simulink model "PE_test"  (R2022b)
settings: Solver=FixedStepAuto  StartTime=0.0  StopTime=50000  FixedStep=0.05  RelTol=1e-13
values from neighbouring files (symbols this model uses):
  A0 = angle2dcm(E1-0.5,E2+0.8,E3+0.3,'ZXY')    [Pointing_tuning.m]
  n = sqrt(settings.mu/settings.a^3)    [Pointing_tuning.m]    (also in control_tuning.m)
undefined symbols (not defined in the file or in its folder): DiscIntNeverNeededParam, environment, r0, sat, settings, thruster, v0
libraries: matrix_library x4, vrlib x4, cstblocks x2
settings Model: SimulationMode=accelerator  Creator=robertopistonenascone  LastModifiedBy=brent

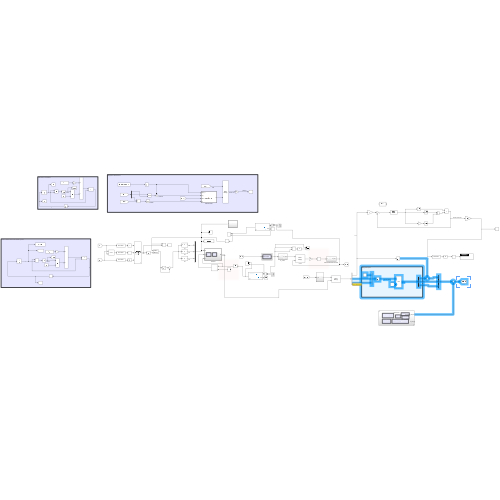
[thumbnail: Simulink's stored preview of the top-level diagram]
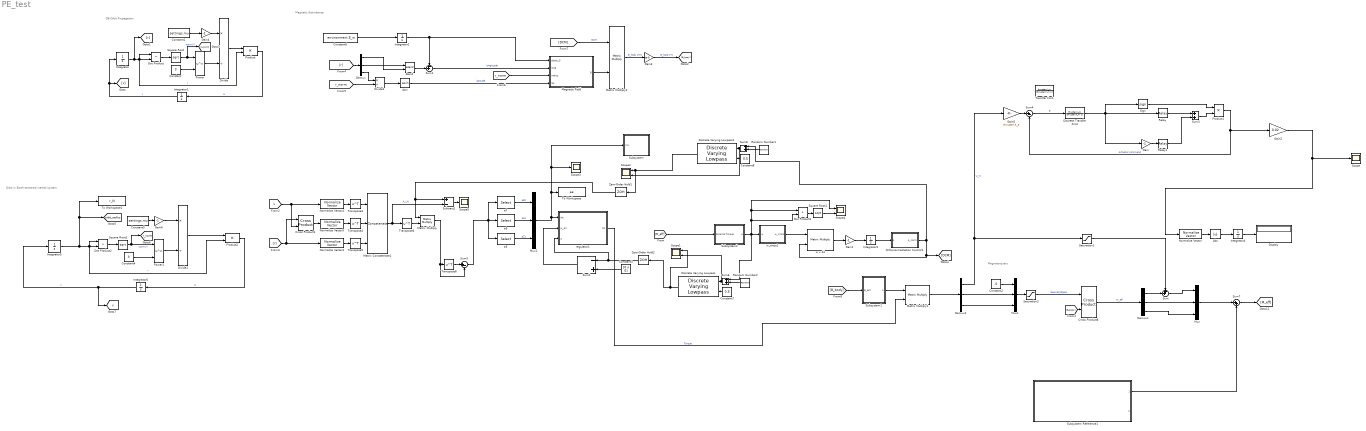
== system PE_test ==
  note: OB Orbit Propagation
  note: Magnetorquers
  note: Magnetic disturbance
  note: Orbit in Earth-centered inertial system
  " w x A1" : Product  Multiplication=Matrix(*)
  Abs : Abs  SaturateOnIntegerOverflow=off
  Asin : Trigonometry  Operator=asin
  Atan2 : Trigonometry  Operator=atan2
  Constant : Constant  Value=3
  Constant1 : Constant  Value=settings.mu
  Constant2 : Constant  Value=0
  Constant3 : Constant  Value=[0 n 0]
  Constant4 : Constant  Value=3
  Constant5 : Constant  Value=settings.mu
  Constant6 : Constant  Value=environment.E_w
  Constant7 : Constant  Value=0.5
  Constant8 : Constant  Value=0.5
  Cross Product1 : matrix_library/Cross Product
  Cross Product8 : matrix_library/Cross Product
  Demux : Demux  Outputs=3
  Demux1 : Demux  Outputs=3
  Demux2 : Demux  Outputs=3
  Discrete Transfer Fcn2 : DiscreteTransferFcn  Numerator=thruster.K_m  Denominator=[thruster.T_m 1]  SampleTime=0.05
  Discrete Varying Lowpass : cstblocks/Linear Parameter Varying/Discrete Varying Lowpass  N=1  w0=0  Ts=0.05
  Discrete Varying Lowpass1 : cstblocks/Linear Parameter Varying/Discrete Varying Lowpass  N=1  w0=0  Ts=0.05
  Display : Display
  Divide : Product  Inputs=*/
  Divide1 : Product  Inputs=*/
  Divide2 : Product  Inputs=*/
  Dot Product : DotProduct  OutDataTypeStr=Inherit: Inherit via internal rule
  Dot Product1 : DotProduct  OutDataTypeStr=Inherit: Inherit via internal rule
  Dot Product2 : DotProduct  OutDataTypeStr=Inherit: Inherit via internal rule
  Gain{,1,4,6} (4 alike) : Gain  Gain=-1
  Gain2 : Gain  Gain=0.02
  Gain3 : Gain  Gain=1e-9
  Gain5 : Gain  Gain=thruster.K_e
  Integrator : Integrator  InitialCondition=r0
  Integrator1 : Integrator  InitialCondition=v0
  Integrator2 : Integrator  InitialCondition=environment.theta_G0
  Integrator3 : Integrator  InitialCondition=A0
  Integrator4 : Integrator
  Integrator5 : Integrator  InitialCondition=r0
  Integrator6 : Integrator  InitialCondition=v0
  Magnetic Field : MATLAB Function  TreatAsAtomicUnit=on
  Matrix Concatenate1 : Concatenate  NumInputs=3  Mode=Multidimensional array
  Matrix Multiply : Product  Multiplication=Matrix(*)
  Matrix Multiply1 : Product  Multiplication=Matrix(*)
  Matrix Multiply2 : Product  Multiplication=Matrix(*)
  Mux : Mux  Inputs=3
  Mux1 : Mux  Inputs=3
  Mux2 : Mux  Inputs=3
  Normalize Vector{,3..5} (4 alike) : vrlib/Utilities/Normalize Vector  maxzero=0
  Orthonormalization Control1 : Subsystem
  Power : Math  Operator=pow
  Power1 : Math  Operator=pow
  Product : Product
  Product1 : Product
  Product2 : Product
  Random Number1 : RandomNumber  Variance=1e-10  SampleTime=0.05
  Random Number2 : RandomNumber  Variance=1e-10  SampleTime=0.05
  Relay : Relay  OnSwitchValue=thruster.Uon  OffSwitchValue=thruster.Uoff
  Relay1 : Relay  OnSwitchValue=thruster.Uon  OffSwitchValue=thruster.Uoff
  Saturation1 : Saturate  UpperLimit=0.02  LowerLimit=-0.02
  Saturation2 : Saturate  UpperLimit=300  LowerLimit=-300
  Scope : Scope
  Scope1 : Scope  NumInputPorts=2
  Scope2 : Scope  NumInputPorts=2
  Scope3 : Scope
  Scope4 : Scope  NumInputPorts=2
  Scope5 : Scope
  Sign : Signum
  Square Root : Sqrt
  Square Root1 : Sqrt
  Square Root2 : Sqrt
  Subsystem : Subsystem  TreatAsAtomicUnit=on  SystemSampleTime=1
  Subsystem Reference1 : Subsystem  ReferencedSubsystem=Enviroment
  Subsystem1 : Subsystem
  Subsystem2 : Subsystem
  Subtract1 : Sum  Inputs=+-
  Sum : Sum  Inputs=++|
  Sum1 : Sum  Inputs=-+|
  Sum2 : Sum  Inputs=-+
  Sum3 : Sum
  Sum4 : Sum  Inputs=|+-
  Sum5 : Sum  Inputs=|+-
  Sum6 : Sum
  Sum7 : Sum  Inputs=|++
  Sum8 : Sum
  To Workspace : ToWorkspace  VariableName=ae  SampleTime=-1
  To Workspace1 : ToWorkspace  VariableName=r_N  SampleTime=-1
  Transfer Fcn1 : TransferFcn  Numerator=thruster.K_m  Denominator=[thruster.T_m 1]
  Transpose{3..6,8} (5 alike) : Math  Operator=transpose
  Zero-Order Hold1 : ZeroOrderHold
  Zero-Order Hold2 : ZeroOrderHold
  a5 : Selector  NumberOfDimensions=2  InputPortWidth=3  IndexOptions=Index vector (dialog),Index vector (dialog)  Indices=2,1  OutputSizes=1,1
  a7 : Selector  NumberOfDimensions=2  InputPortWidth=3  IndexOptions=Index vector (dialog),Index vector (dialog)  Indices=3,2  OutputSizes=1,1
  a9 : Selector  NumberOfDimensions=2  InputPortWidth=3  IndexOptions=Index vector (dialog),Index vector (dialog)  Indices=1,3  OutputSizes=1,1
  regulator1 : Subsystem  TreatAsAtomicUnit=on  SystemSampleTime=1
  w_cross1 : Subsystem
  tag scope: orbit_radius=global, r_norm=global, v=global
  wires:
  Gain3/1 -> [B_body]  "B_body [T]"
  Demux1/2 -> Mux/2
  Demux1/1 -> Sum/2
  [M_eff] -> Subsystem2/1(External Torque)
  Demux/2 -> Atan2/1
  Constant2/1 -> Mux1/1
  Constant6/1 -> Integrator2/1
  Normalize Vector5/1 -> Transpose4/1
  Mux1/1 -> Saturation2/1
  Matrix Multiply1/1 -> Demux2/1
  Demux2/3 -> Mux1/3
  w_cross1/1(w_cross) -> " w x A1"/1
  [r_norm] -> Divide2/2
  Sum/1 -> Mux/1
  Matrix Multiply/1 -> Sum5/2, Transpose8/1
  Transpose5/1 -> Matrix Concatenate1/3
  Demux1/3 -> Mux/3
  Integrator1/1 -> [v], Integrator/1  "v"
  Normalize Vector4/1 -> Transpose3/1
  a9/1 -> Mux2/2  "a13"
  [DCM] -> Matrix Multiply2/1  "DCM"
  [r] -> Demux/1
  Integrator2/1 -> Sum1/1, Magnetic Field/1(alpha_G)
  Demux/3 -> Divide2/1
  Dot Product1/1 -> Square Root1/1
  Demux/1 -> Atan2/2
  Sum1/1 -> Magnetic Field/2(long)  "longitutde"
  Atan2/1 -> Sum1/2
  [B_body] -> Cross Product8/2
  Matrix Multiply2/1 -> Gain3/1  "B_body [nT]"
  Transpose6/1 -> Matrix Multiply/2
  Divide2/1 -> Asin/1
  Transpose3/1 -> Matrix Concatenate1/1
  Cross Product1/1 -> Normalize Vector5/1
  Matrix Concatenate1/1 -> Subtract1/2, Transpose6/1  "A_LN"
  regulator1/1(Mc) -> Matrix Multiply1/2  "Torque"
  [v] -> Normalize Vector4/1, Cross Product1/2
  Constant/1 -> Power/2
  [B_body] -> Subsystem1/1(B_est)
  Gain4/1 -> Divide/1
  Transpose4/1 -> Matrix Concatenate1/2
  Magnetic Field/1(B) -> Matrix Multiply2/2
  Transpose8/1 -> Sum5/1
  [r] -> Cross Product1/1, Normalize Vector3/1
  Sum2/1 -> regulator1/2(w_err)
  Constant1/1 -> Gain4/1
  Demux2/2 -> Mux1/2
  Normalize Vector3/1 -> Transpose5/1
  Integrator3/1 -> Orthonormalization Control1/1(A)
  Asin/1 -> Magnetic Field/4(lat)  "latitude"
  a5/1 -> Mux2/3  "a21"
  Cross Product8/1 -> Demux1/1  "M_eff"
  Gain1/1 -> Integrator3/1
  Integrator/1 -> [r], Product/2, Dot Product/2, Dot Product/1  "r"
  " w x A1"/1 -> Gain1/1
  Mux2/1 -> To Workspace/1, Subsystem/1(In1), Scope3/1, regulator1/1(Ae)
  [r_norm] -> Magnetic Field/3(radius)
  Constant3/1 -> Sum2/2
  Dot Product/1 -> Square Root/1
  Subsystem1/1(A) -> Matrix Multiply1/1
  Divide/1 -> Product/1
  Product/1 -> Integrator1/1  "a"
  a7/1 -> Mux2/1  "a32"
  Sum5/1 -> a5/1, a9/1, a7/1
  Power/1 -> Divide/2
  Square Root/1 -> [r_norm], Power/1  "norm(r)"
  Square Root1/1 -> Scope4/2
  Abs/1 -> Integrator4/1
  Integrator4/1 -> Display/1
  Normalize Vector/1 -> Abs/1
  Gain2/1 -> Scope/1, Normalize Vector/1
  Demux2/1 -> Saturation1/1, Gain5/1  "U_in"
  Sign/1 -> Product1/1
  Relay/1 -> Sum3/1
  Sum3/1 -> Product1/2
  Product1/1 -> Gain2/1, Sum4/2  "Actuator command"
  Gain5/1 -> Sum4/1
  Sum4/1 -> Discrete Transfer Fcn2/1  "E"
  Gain/1 -> Relay1/1
  Relay1/1 -> Sum3/2
  Discrete Transfer Fcn2/1 -> Relay/1, Sign/1, Gain/1
  Saturation2/1 -> Cross Product8/1  "required dipole"
  Sum7/1 -> [M_eff]
  Subsystem Reference1/1 -> Sum7/2
  Divide1/1 -> Product2/1
  Integrator5/1 -> [orbit_radius], To Workspace1/1, Product2/2, Dot Product2/2, Dot Product2/1  "r"
  Square Root2/1 -> [r_norm], Power1/1  "norm(r)"
  Constant4/1 -> Power1/2
  Dot Product2/1 -> Square Root2/1
  Constant5/1 -> Gain6/1
  Power1/1 -> Divide1/2
  Gain6/1 -> Divide1/1
  Product2/1 -> Integrator6/1  "a"
  Integrator6/1 -> Integrator5/1, [v]  "v"
  Subsystem2/1(w) -> Sum6/1, Scope4/1, Dot Product1/1, Dot Product1/2, w_cross1/1(w)
  Random Number2/1 -> Sum6/2
  Zero-Order Hold1/1 -> Subtract1/1, Matrix Multiply/1
  Zero-Order Hold2/1 -> Sum2/1, regulator1/3(w)
  Sum6/1 -> Scope1/2, Discrete Varying Lowpass/1
  Constant7/1 -> Discrete Varying Lowpass/2
  Discrete Varying Lowpass/1 -> Scope1/1, Zero-Order Hold2/1
  Constant8/1 -> Discrete Varying Lowpass1/2
  Sum8/1 -> Scope2/2, Discrete Varying Lowpass1/1
  Random Number1/1 -> Sum8/2
  Orthonormalization Control1/1(A_norm) -> [DCM], " w x A1"/2, Sum8/1
  Discrete Varying Lowpass1/1 -> Zero-Order Hold1/1, Scope2/1
  Subtract1/1 -> Scope5/1
  Mux/1 -> Sum7/1
  Saturation1/1 -> Sum/1

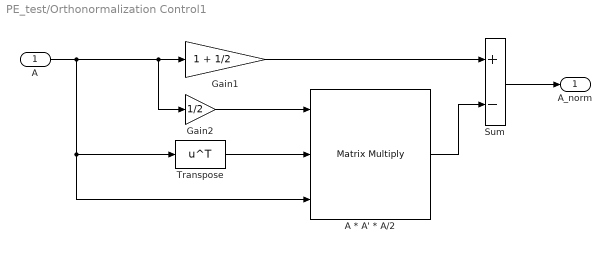
== system PE_test/Orthonormalization Control1 ==
  A : Inport
  " A * A' * A/2" : Product  Inputs=3  Multiplication=Matrix(*)
  Gain1 : Gain  Gain=1 + 1/2
  Gain2 : Gain  Gain=1/2
  Sum : Sum  Inputs=+-
  Transpose : Math  Operator=transpose
  A_norm : Outport
  wires:
  A/1 -> Transpose/1, " A * A' * A/2"/3, Gain1/1, Gain2/1
  Gain1/1 -> Sum/1
  " A * A' * A/2"/1 -> Sum/2
  Sum/1 -> A_norm/1
  Gain2/1 -> " A * A' * A/2"/1
  Transpose/1 -> " A * A' * A/2"/2

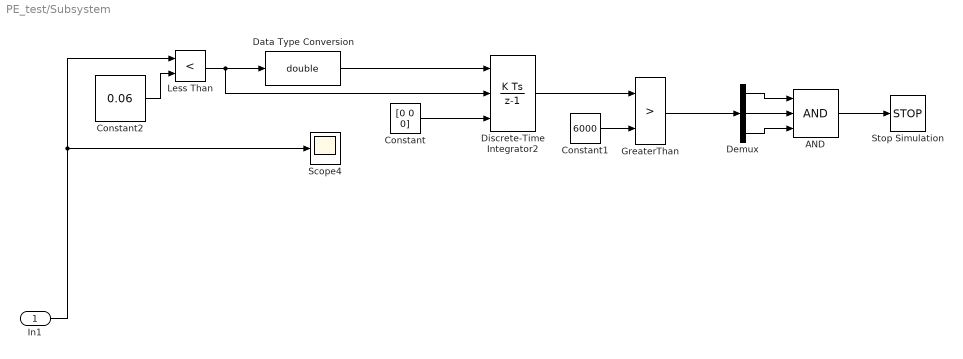
== system PE_test/Subsystem ==
  In1 : Inport
  AND : Logic  Inputs=3  IconShape=distinctive  AllPortsSameDT=off  OutDataTypeStr=boolean
  Constant : Constant  Value=[0 0 0]
  Constant1 : Constant  Value=6000
  Constant2 : Constant  Value=0.06
  Data Type Conversion : DataTypeConversion  OutDataTypeStr=double  SaturateOnIntegerOverflow=off  RndMeth=Floor
  Demux : Demux  Outputs=3
  Discrete-Time Integrator2 : DiscreteIntegrator  ExternalReset=either  InitialConditionSource=external  ICPrevOutput=DiscIntNeverNeededParam  ICPrevScaledInput=DiscIntNeverNeededParam
  GreaterThan : RelationalOperator  Operator=>  OutDataTypeStr=boolean  RndMeth=Simplest  InputSameDT=off
  Less Than : RelationalOperator  Operator=<  OutDataTypeStr=boolean  RndMeth=Simplest  InputSameDT=off
  Scope4 : Scope
  Stop Simulation : Stop
  wires:
  Data Type Conversion/1 -> Discrete-Time Integrator2/1
  Less Than/1 -> Discrete-Time Integrator2/2, Data Type Conversion/1
  In1/1 -> Scope4/1, Less Than/1
  Constant2/1 -> Less Than/2
  Discrete-Time Integrator2/1 -> GreaterThan/1
  Constant/1 -> Discrete-Time Integrator2/3
  Constant1/1 -> GreaterThan/2
  GreaterThan/1 -> Demux/1
  Demux/2 -> AND/2
  Demux/3 -> AND/3
  Demux/1 -> AND/1
  AND/1 -> Stop Simulation/1

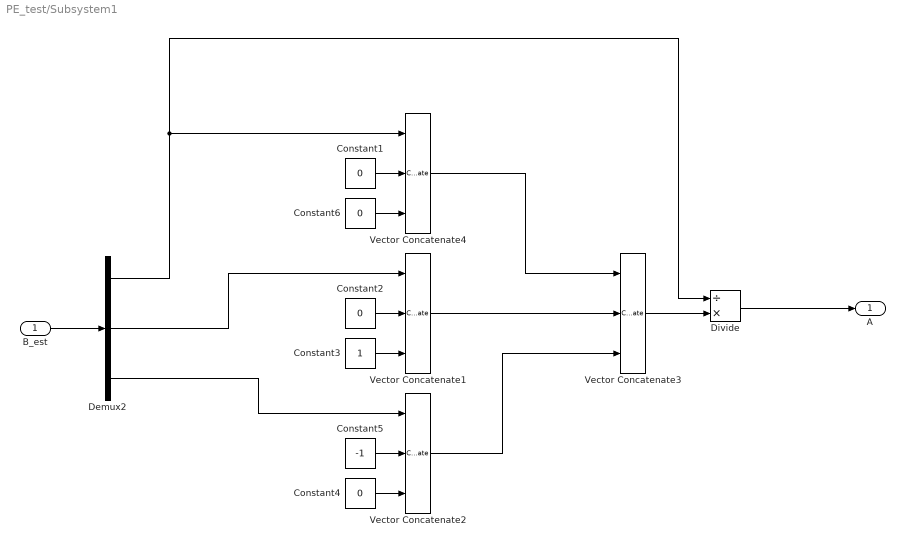
== system PE_test/Subsystem1 ==
  B_est : Inport
  Constant{1..2,4,6} (4 alike) : Constant  Value=0
  Constant3 : Constant
  Constant5 : Constant  Value=-1
  Demux2 : Demux  Outputs=3
  Divide : Product  Inputs=/*
  Vector Concatenate1 : Concatenate  NumInputs=3  Mode=Multidimensional array
  Vector Concatenate2 : Concatenate  NumInputs=3  Mode=Multidimensional array
  Vector Concatenate3 : Concatenate  NumInputs=3  Mode=Multidimensional array  ConcatenateDimension=2
  Vector Concatenate4 : Concatenate  NumInputs=3  Mode=Multidimensional array
  A : Outport
  wires:
  Vector Concatenate1/1 -> Vector Concatenate3/2
  B_est/1 -> Demux2/1
  Vector Concatenate4/1 -> Vector Concatenate3/1
  Demux2/2 -> Vector Concatenate1/1
  Constant2/1 -> Vector Concatenate1/2
  Constant3/1 -> Vector Concatenate1/3
  Constant5/1 -> Vector Concatenate2/2
  Constant4/1 -> Vector Concatenate2/3
  Demux2/3 -> Vector Concatenate2/1
  Vector Concatenate2/1 -> Vector Concatenate3/3
  Demux2/1 -> Divide/1, Vector Concatenate4/1
  Vector Concatenate3/1 -> Divide/2
  Divide/1 -> A/1
  Constant1/1 -> Vector Concatenate4/2
  Constant6/1 -> Vector Concatenate4/3

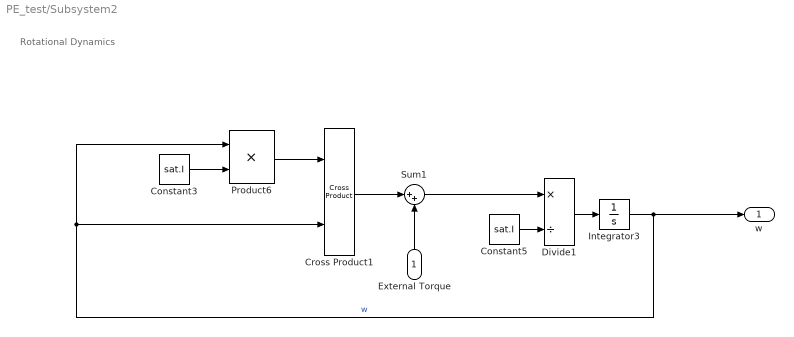
== system PE_test/Subsystem2 ==
  note: Rotational Dynamics
  External Torque : Inport
  Constant3 : Constant  Value=sat.I
  Constant5 : Constant  Value=sat.I
  Cross Product1 : matrix_library/Cross Product
  Divide1 : Product  Inputs=*/
  Integrator3 : Integrator  InitialCondition=settings.w0
  Product6 : Product
  Sum1 : Sum  Inputs=|++
  w : Outport
  wires:
  Constant5/1 -> Divide1/2
  Sum1/1 -> Divide1/1
  External Torque/1 -> Sum1/2
  Integrator3/1 -> w/1, Cross Product1/2, Product6/1  "w"
  Divide1/1 -> Integrator3/1
  Cross Product1/1 -> Sum1/1
  Constant3/1 -> Product6/2
  Product6/1 -> Cross Product1/1

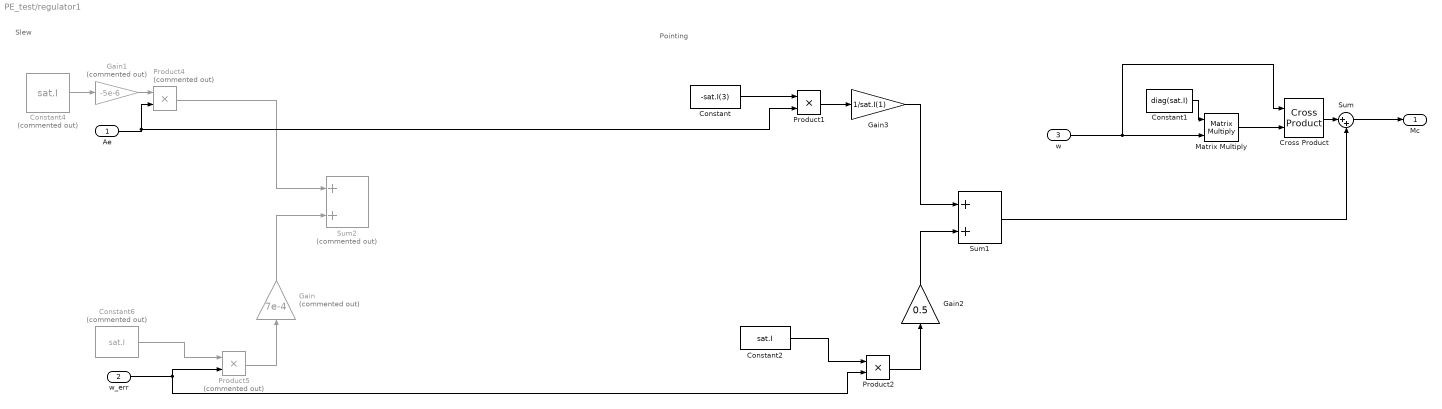
== system PE_test/regulator1 ==
  note: Slew
  note: Pointing
  Ae : Inport
  w_err : Inport  Port=2
  w : Inport  Port=3
  Constant : Constant  Value=-sat.I(3)
  Constant1 : Constant  Value=diag(sat.I)
  Constant2 : Constant  Value=sat.I
  Constant4 : Constant  Commented=on  Value=sat.I
  Constant6 : Constant  Commented=on  Value=sat.I
  Cross Product : matrix_library/Cross Product
  Gain : Gain  Commented=on  Gain=7e-4
  Gain1 : Gain  Commented=on  Gain=-5e-6
  Gain2 : Gain  Gain=0.5
  Gain3 : Gain  Gain=1/sat.I(1)
  Matrix Multiply : Product  Multiplication=Matrix(*)
  Product1 : Product
  Product2 : Product
  Product4 : Product  Commented=on
  Product5 : Product  Commented=on
  Sum : Sum  Inputs=|++
  Sum1 : Sum
  Sum2 : Sum  Commented=on
  Mc : Outport
  wires:
  Product5/1 -> Gain/1
  Constant6/1 -> Product5/1
  Gain/1 -> Sum2/2
  Gain1/1 -> Product4/1
  Constant4/1 -> Gain1/1
  Constant/1 -> Product1/1
  Gain2/1 -> Sum1/2
  Constant2/1 -> Product2/1
  Product2/1 -> Gain2/1
  Product1/1 -> Gain3/1
  Product4/1 -> Sum2/1
  Gain3/1 -> Sum1/1
  Ae/1 -> Product1/2, Product4/2
  w_err/1 -> Product2/2, Product5/2
  w/1 -> Matrix Multiply/2, Cross Product/1
  Constant1/1 -> Matrix Multiply/1
  Matrix Multiply/1 -> Cross Product/2
  Cross Product/1 -> Sum/1
  Sum/1 -> Mc/1
  Sum1/1 -> Sum/2

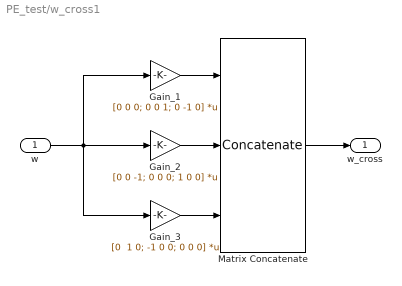
== system PE_test/w_cross1 ==
  w : Inport
  Gain_1 : Gain  Gain=[0 0 0; 0 0 1; 0 -1 0]  Multiplication=Matrix(K*u)
  Gain_2 : Gain  Gain=[0 0 -1; 0 0 0; 1 0 0]  Multiplication=Matrix(K*u)
  Gain_3 : Gain  Gain="[0  1 0; -1 0 0; 0 0 0]"  Multiplication=Matrix(K*u)
  Matrix Concatenate : Concatenate  NumInputs=3  Mode=Multidimensional array  ConcatenateDimension=2
  w_cross : Outport
  wires:
  w/1 -> Gain_2/1, Gain_1/1, Gain_3/1
  Gain_3/1 -> Matrix Concatenate/3
  Gain_2/1 -> Matrix Concatenate/2
  Gain_1/1 -> Matrix Concatenate/1
  Matrix Concatenate/1 -> w_cross/1

== matlab function PE_test/Magnetic Field ==
  data: alpha_G input; long input; radius input; B output; lat input; environment parameter; settings parameter
function B = magneticField(alpha_G,long,radius,lat,environment,settings)
%{  
    Return the magnetic field component in inertial reference frame

%}
theta = (pi/2-lat);     % theta is the colatitude [rad]
alpha = long + alpha_G; 

g = environment.WMM.g;
h = environment.WMM.h;
K = environment.WMM.K;
R = environment.R;
N = settings.N;

%% P-dP
% validated through the P and dP tables in "Jeremy Davis, Mathematical Modeling of Earthas Magnetic
% Field, 2004"

%%%%%%%%%%%%%%%%%%%%%%%%%%%%%%%%%%%%%%%%%%%%%%%%%%%%%%%%%%%%%%%%%%%%%%%%%%%%%%%%%%%%%%%%%%%%%%%%
% P_{(n),(m+1)}: 
% given P(a,b) -> n=a, m=b-1
% n from 1 to N
% m from 0 to N
% N order of accuracy
%%%%%%%%%%%%%%%%%%%%%%%%%%%%%%%%%%%%%%%%%%%%%%%%%%%%%%%%%%%%%%%%%%%%%%%%%%%%%%%%%%%%%%%%%%%%%%%%

P = zeros(N,N+1);
dP = zeros(N,N+1);

P_00 = 1;
dP_00 = 0;

P_01 = 0; 
dP_01 = 0;

P(1,1) = cos(theta); % n=1, m=0
dP(1,1) = -sin(theta)*P_00; 

P(1,2) = sin(theta);  % n=1, m=1
dP(1,2) = cos(theta)*P_00;

for i = 2:N % ciclo in n a partire da n=2 a n=N
    for j = 0:i % ciclo in m da m=0 a m=n
        if j == i
        P(i,j+1) = sin(theta)*P(i-1,j);
        dP(i,j+1) = sin(theta)*dP(i-1,j) + cos(theta)*P(i-1,j);
        elseif i < 3
            if j == 0 % n=2, m=0
            P(i,j+1) = cos(theta)*P(i-1,j+1) - K(i,j+1)*P_00;
            dP(i,j+1) = -sin(theta)*P(i-1,j+1) + cos(theta)*dP(i-1,j+1) ...
                - K(i,j+1)*dP_00;
            elseif j == 1 % n=2, m=1
                P(i,j+1) = cos(theta)*P(i-1,j+1) - K(i,j+1)*P_01;
                dP(i,j+1) = -sin(theta)*P(i-1,j+1) + cos(theta)*dP(i-1,j+1)...
                    - K(i,j+1)*dP_01;
            end
        else
            P(i,j+1) = cos(theta)*P(i-1,j+1) - K(i,j+1)*P(i-2,j+1);
            dP(i,j+1) = -sin(theta)*P(i-1,j+1) + cos(theta)*dP(i-1,j+1) ...
                - K(i,j+1)*dP(i-2,j+1);
        end
    end
end

%% Magnetic Field

B_r = 0;
B_th = 0;
B_phi = 0;

%indice i scorre n da 1 a N
%indice j scorre m da 0 a n

for m = 0:N
    for n = 1:N
        if m<=n
            B_r = B_r + (R/radius)^(n+2)*(n+1)*...
                ((g(n,m+1)*cos(m*long) + h(n,m+1)*sin(m*long))*P(n, m+1));
            B_th = B_th + (R/radius)^(n+2)*...
                ((g(n,m+1)*cos(m*long) + h(n,m+1)*sin(m*long))*dP(n, m+1));
            B_phi = B_phi + (R/radius)^(n+2)*...
                (m*(-g(n,m+1)*sin(m*long) + h(n,m+1)*cos(m*long))* P(n, m+1));

        end

    end
end

B_th = -B_th;
B_phi = -B_phi/sin(theta);

B_x = ( B_r*cos(lat) + B_th*sin(lat) ) * cos(alpha) - B_phi*sin(alpha);
B_y = ( B_r*cos(lat) + B_th*sin(lat) ) * sin(alpha) + B_phi*cos(alpha);
B_z = B_r*sin(lat) + B_th*cos(lat);

B = [B_x B_y B_z]';
